simulink model "bh_solenoid_simscape_FINAL"  (R2018a)
settings: Solver=VariableStepAuto  StartTime=0.0  StopTime=3  MaxStep=0.01  RelTol=1e-3  AbsTol=1e-3  EnableMultiTasking=on
undefined symbols (not defined in the file): Coeffs, Elec, Mech, sigbuilder_block, solen
libraries: fl_lib x16, nesl_utility x7
CloseFcn:
  | try,close(h1_ssc_solenoid),end
  | clear h1_ssc_solenoid
  | 
  | clear simlog_ssc_solenoid
Description:
  | Solenoid
  | 
  | Copyright 2008-2017 The MathWorks, Inc.
settings Model: Creator=MathWorks  LastModifiedBy=bhorton
settings SolverCC: AutoScaleAbsTol=off
settings DataIOCC: LimitDataPoints=on  SaveFormat=Array
settings OptimizationCC: LifeSpan=inf
settings DebuggingCC: SolverPrmCheckMsg=warning  AllowSymbolicDim=off  SFUnexpectedBacktrackingDiag=warning  SFNoUnconditionalDefaultTransitionDiag=warning  SFExecutionAtInitializationDiag=none
settings HardwareCC: ProdBitPerPointer=32  ProdBitPerSizeT=32  ProdBitPerPtrDiffT=32  ProdLargestAtomicFloat=None  ProdIntDivRoundTo=Undefined  ProdEndianess=Unspecified  ProdWordSize=32  ProdHWDeviceType=32-bit Generic
settings ModelReferenceCC: PropagateSignalLabelsOutOfModel=off
settings CodeAppCC: StateflowObjectComments=on
settings GRTTargetCC: TargetLangStandard=C89/C90 (ANSI)  GeneratePreprocessorConditionals=Disable all
settings ConfigComp: CovMetricSettings=dw  CovHtmlReporting=on  CovSaveCumulativeToWorkspaceVar=on  CovSaveSingleToWorkspaceVar=on  CovExternalEMLEnable=off  CovSFcnEnable=off
settings SimscapeCC: SimscapeLogType=all  SimscapeLogSimulationStatistics=on  SimscapeLogName=simlog_ssc_solenoid  SimscapeLogDataHistory=10000

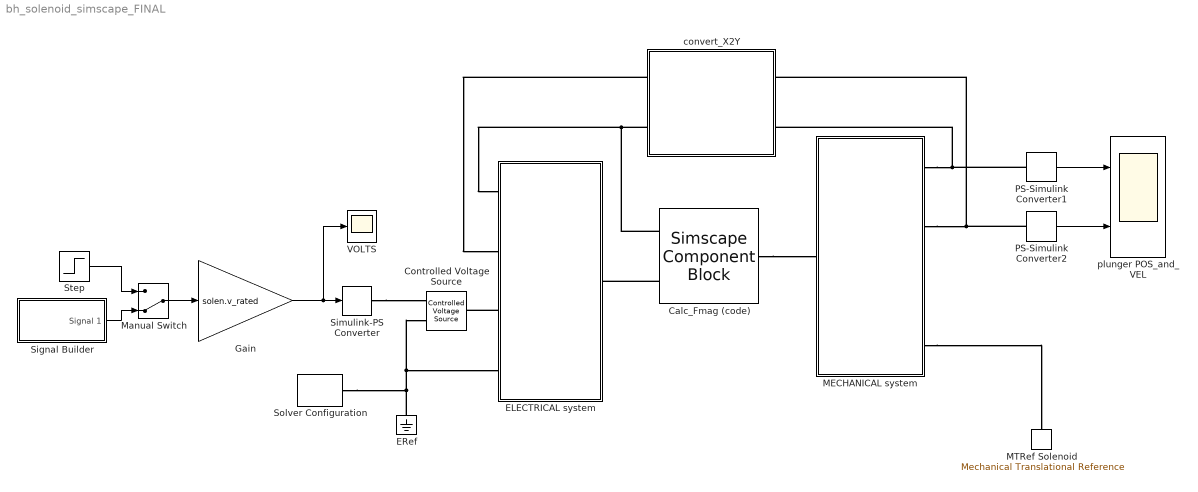
== system bh_solenoid_simscape_FINAL ==
  Calc_Fmag (code) : SimscapeComponentBlock  SourceFile=bh_Fmag  ComponentPath=bh_Fmag  ComponentVariants=bh_Fmag  ComponentVariantNames=bh_Fmag  ClassName=bh_Fmag  SchemaVersion=1  C1=Coeffs.C123(1) m^5*H  C2=Coeffs.C123(2) m^2  C3=Coeffs.C123(3) m^3
      settings: CopyFcn=simscape.engine.sli.internal.componentblockcallback(gcbh,'COPY')  PreCopyFcn=simscape.engine.sli.internal.componentblockcallback(gcbh,'PRECOPY')  PreDeleteFcn=simscape.engine.sli.internal.componentblockcallback(gcbh,'PREDELETE')
      mask Type: bh_Fmag
      mask Display:
      | disp('Simscape\n\n\n')
      | disp('\n\n\nbh_Fmag');
      | color('red');
      | port_label('RConn', 1,'Fmag');
      | port_label('LConn', 2,'i');
      | port_label('LConn', 1,'Y');
  Controlled Voltage Source : fl_lib/Electrical/Electrical Sources/Controlled Voltage Source
  ELECTRICAL system : Subsystem
  ERef : fl_lib/Electrical/Electrical Elements/Electrical Reference
  Gain : Gain  Gain=solen.v_rated
  MECHANICAL system : Subsystem
  MTRef Solenoid : fl_lib/Mechanical/Translational Elements/Mechanical Translational Reference
  Manual Switch : ManualSwitch  CurrentSetting=0
  PS-Simulink Converter1 : nesl_utility/PS-Simulink Converter  PhysicalDomain=network_engine_domain  SubClassName=ps_output  LeftPortType=input  RightPortType=output  PseudoPeriodic=off  Frequencies=[]  Unit=m  AffineConversion=off
      settings: AttributesFormatString=units=%<Unit>
  PS-Simulink Converter2 : nesl_utility/PS-Simulink Converter  PhysicalDomain=network_engine_domain  SubClassName=ps_output  LeftPortType=input  RightPortType=output  PseudoPeriodic=off  Frequencies=[]  Unit=m/s  AffineConversion=off
      settings: AttributesFormatString=units=%<Unit>
  Signal Builder : Subsystem  Tag=STV Subsys  LoadFcn=sigbuilder_block('load');  StartFcn=sigbuilder_block('start');  StopFcn=sigbuilder_block('stop');  ClipboardFcn=sigbuilder_block('clipboard');  mask(Sigbuilder block){tuvar=[0:10]}
      mask help: Simulink:masks:SigbuilderBlock_MD
      mask init:
      | if ~strcmp(get_param(bdroot(gcbh),'SimulationStatus'),'stopped') tuvar = sigbuilder_block('maskInit'); end
      settings: CopyFcn=sigbuilder_block('copy');  DeleteFcn=sigbuilder_block('delete');  ModelCloseFcn=sigbuilder_block('modelClose');  PreSaveFcn=sigbuilder_block('preSave');  PauseFcn=sigbuilder_block('pause');  ContinueFcn=sigbuilder_block('continue');  NameChangeFcn=sigbuilder_block('namechange');  OpenFcn=sigbuilder_block('open',[437.6 199.2 550.4 400 ]);  CloseFcn=sigbuilder_block('close');
      mask Display: plot(0, 0, 100, 100,[2, 2, 32, 32, 2], [68, 8, 8, 68, 68],[32, 2], [38, 38], [32, 19, 2],[53, 60, 44], [32, 17, 17, 2],[16, 16, 31, 31]);txt = getActiveGroup(gcbh);text(2, 100, txt,'verticalAlignment', 'top');
  Simulink-PS Converter : nesl_utility/Simulink-PS Converter  PhysicalDomain=network_engine_domain  SubClassName=ps_input  LeftPortType=input  RightPortType=output  PseudoPeriodic=off  Frequencies=[]  NoiseDistribution=none  NoiseParameters=[]  Unit=V  AffineConversion=off  FilteringAndDerivatives=provide  SimscapeFilterOrder=1  InputFilterTimeConstant=0.001  UdotUserProvided=0
  Solver Configuration : nesl_utility/Solver Configuration  PhysicalDomain=network_engine_domain  SubClassName=solver  LeftPortType=input  RightPortType=generic  Tones=[]  Harmonics=[]  SimulateNoise=off  Profile=off  UseLocalSampling=off  EnableSwitchedLinearOptims=on  FrequencyDomain=off  UseCCode=off  RelTol=0.001  AbsTol=1e-06  MinStep=1e-09  ToWorkspace=off  RevertToSquareIcSolve=off  NumHomotopyIterations=100  PhasorMode=off  PhasorModeNumHarmonics=1  DoDC=off  ResidualTolerance=1e-09  UseLocalSolver=off  LocalSolverChoice=NE_BACKWARD_EULER_ADVANCER  LocalSolverSampleTime=0.001  DoFixedCost=off  MaxNonlinIter=3  MaxModeIter=2  LinearAlgebra=Sparse  EquationFormulation=NE_TIME_EF  DelaysMemoryBudget=1024  AutomaticFiltering=on  FilteringTimeConstant=0.001
  Step : Step  Time=0.1  SampleTime=0
  VOLTS : Scope
  convert_X2Y : Subsystem
  plunger POS_and_VEL : Scope  NumInputPorts=2
  wires:
  Signal Builder/1(Signal 1) -> Manual Switch/2
  Manual Switch/1 -> Gain/1
  Step/1 -> Manual Switch/1
  Gain/1 -> VOLTS/1, Simulink-PS Converter/1
  PS-Simulink Converter1/1 -> plunger POS_and_VEL/1
  PS-Simulink Converter2/1 -> plunger POS_and_VEL/2
  connections:
  ELECTRICAL system/LConn3 -- Controlled Voltage Source/LConn1
  ERef/LConn1 -- Controlled Voltage Source/RConn2 -- ELECTRICAL system/LConn4 -- Solver Configuration/RConn1
  Simulink-PS Converter/RConn1 -- Controlled Voltage Source/RConn1
  MECHANICAL system/RConn1 -- PS-Simulink Converter1/LConn1 -- convert_X2Y/LConn2
  MECHANICAL system/RConn2 -- PS-Simulink Converter2/LConn1 -- convert_X2Y/LConn1
  convert_X2Y/RConn1 -- ELECTRICAL system/LConn2
  convert_X2Y/RConn2 -- Calc_Fmag (code)/LConn1 -- ELECTRICAL system/LConn1
  Calc_Fmag (code)/RConn1 -- MECHANICAL system/LConn1
  Calc_Fmag (code)/LConn2 -- ELECTRICAL system/RConn1
  MECHANICAL system/RConn4 -- MTRef Solenoid/LConn1

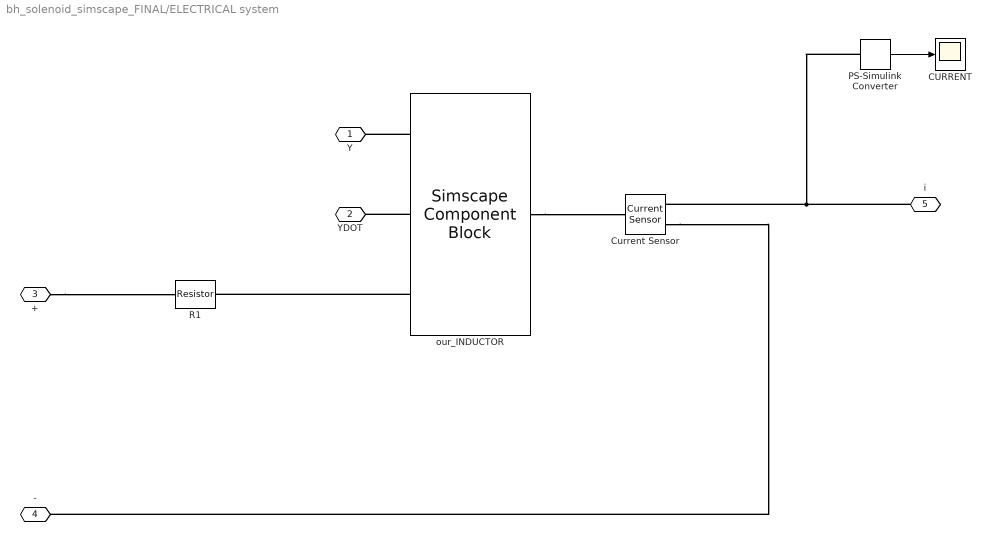
== system bh_solenoid_simscape_FINAL/ELECTRICAL system ==
  CURRENT : Scope
  Current Sensor : fl_lib/Electrical/Electrical Sensors/Current Sensor
  PS-Simulink Converter : nesl_utility/PS-Simulink Converter  PhysicalDomain=network_engine_domain  SubClassName=ps_output  LeftPortType=input  RightPortType=output  PseudoPeriodic=off  Frequencies=[]  Unit=A  AffineConversion=off
      settings: AttributesFormatString=unit=%<Unit>
  R1 : fl_lib/Electrical/Electrical Elements/Resistor  R=Elec.R Ohm  i_specify=off  i_priority=High  i=0 A  i_nominal_specify=off  i_nominal_unit=A  i_nominal_value=1  v_specify=off  v_priority=High  v=0 V  v_nominal_specify=off  v_nominal_unit=V  v_nominal_value=1
      settings: AttributesFormatString=R=%<R>
  our_INDUCTOR : SimscapeComponentBlock  SourceFile=bh_var_L  ComponentPath=bh_var_L  ComponentVariants=bh_var_L  ComponentVariantNames=bh_var_L  ClassName=bh_var_L  SchemaVersion=1  C1=Coeffs.C123(1) m^5*H  C2=Coeffs.C123(2) m^2  C3=Coeffs.C123(3) m^3  i_specify=off  i_priority=None  i=0 A  i_nominal_specify=off  i_nominal_unit=A  i_nominal_value=1  v_specify=off  v_priority=None  v=0 V  v_nominal_specify=off  v_nominal_unit=V  v_nominal_value=1
      settings: CopyFcn=simscape.engine.sli.internal.componentblockcallback(gcbh,'COPY')  PreCopyFcn=simscape.engine.sli.internal.componentblockcallback(gcbh,'PRECOPY')  PreDeleteFcn=simscape.engine.sli.internal.componentblockcallback(gcbh,'PREDELETE')
      mask Type: bh_var_L
      mask Display:
      | disp('Simscape\n\n\n')
      | disp('\n\n\nbh_var_L');
      | color('red');
      | port_label('RConn', 1,'-');
      | port_label('LConn', 3,'+');
      | port_label('LConn', 2,'Y_DOT');
      | port_label('LConn', 1,'Y');
  Y : PMIOPort  Side=Left
  YDOT : PMIOPort  Port=2  Side=Left
  + : PMIOPort  Port=3  Side=Left
  - : PMIOPort  Port=4  Side=Left
  i : PMIOPort  Port=5  Side=Right
  wires:
  PS-Simulink Converter/1 -> CURRENT/1
  connections:
  Current Sensor/RConn2 -- -/RConn1
  +/RConn1 -- R1/LConn1
  i/RConn1 -- PS-Simulink Converter/LConn1 -- Current Sensor/RConn1
  our_INDUCTOR/LConn1 -- Y/RConn1
  our_INDUCTOR/LConn2 -- YDOT/RConn1
  our_INDUCTOR/RConn1 -- Current Sensor/LConn1
  our_INDUCTOR/LConn3 -- R1/RConn1

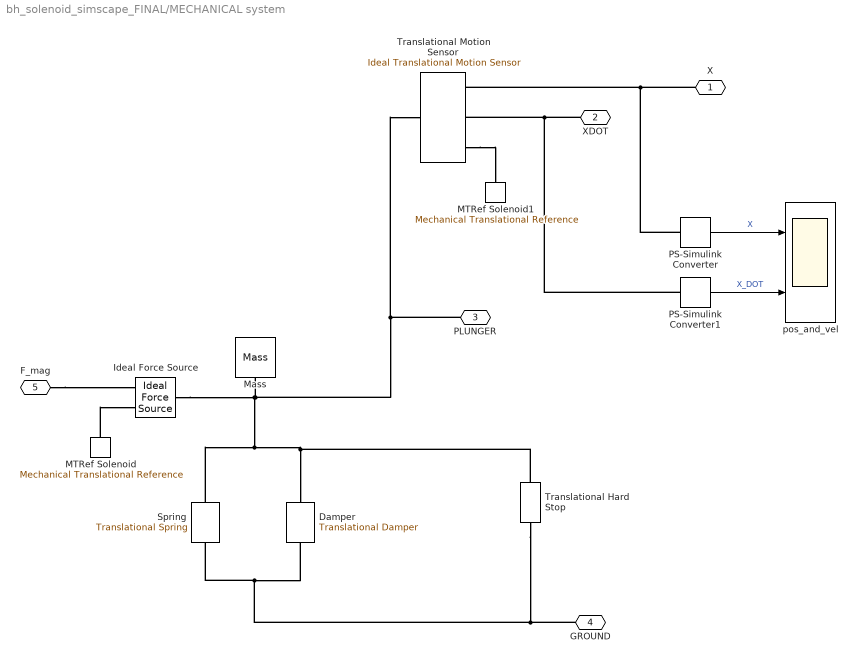
== system bh_solenoid_simscape_FINAL/MECHANICAL system ==
  Damper : fl_lib/Mechanical/Translational Elements/Translational Damper  D=Mech.C N/(m/s)  v_specify=off  v_priority=High  v=0 m/s  v_nominal_specify=off  v_nominal_unit=m/s  v_nominal_value=1  f_specify=off  f_priority=High  f=0 N  f_nominal_specify=off  f_nominal_unit=N  f_nominal_value=1
  Ideal Force Source : fl_lib/Mechanical/Mechanical Sources/Ideal Force Source
  MTRef Solenoid : fl_lib/Mechanical/Translational Elements/Mechanical Translational Reference
  MTRef Solenoid1 : fl_lib/Mechanical/Translational Elements/Mechanical Translational Reference
  Mass : fl_lib/Mechanical/Translational Elements/Mass  mass=Mech.M kg  v_specify=off  v_priority=High  v=0 m/s  v_nominal_specify=off  v_nominal_unit=m/s  v_nominal_value=1  f_specify=off  f_priority=High  f=0 N  f_nominal_specify=off  f_nominal_unit=N  f_nominal_value=1
  PS-Simulink Converter : nesl_utility/PS-Simulink Converter  PhysicalDomain=network_engine_domain  SubClassName=ps_output  LeftPortType=input  RightPortType=output  PseudoPeriodic=off  Frequencies=[]  Unit=m  AffineConversion=off
      settings: AttributesFormatString=unit=%<Unit>
  PS-Simulink Converter1 : nesl_utility/PS-Simulink Converter  PhysicalDomain=network_engine_domain  SubClassName=ps_output  LeftPortType=input  RightPortType=output  PseudoPeriodic=off  Frequencies=[]  Unit=m/s  AffineConversion=off
      settings: AttributesFormatString=unit=%<Unit>
  Spring : fl_lib/Mechanical/Translational Elements/Translational Spring  spr_rate=Mech.K N/m  v_specify=off  v_priority=High  v=0 m/s  v_nominal_specify=off  v_nominal_unit=m/s  v_nominal_value=1  f_specify=off  f_priority=High  f=0 N  f_nominal_specify=off  f_nominal_unit=N  f_nominal_value=1  x_specify=on  x_priority=High  x=Mech.x_0 m  x_nominal_specify=off  x_nominal_unit=m  x_nominal_value=1
      settings: AttributesFormatString=|
      | DEFLECTION=
      | %<x>
  Translational Motion Sensor : fl_lib/Mechanical/Mechanical Sensors/Ideal Translational Motion Sensor  offset=Mech.x_0 m
      settings: AttributesFormatString=|
      | init_VAL =
      | %<offset> %<offset_unit>
  Translational Hard Stop : fl_lib/Mechanical/Translational Elements/Translational Hard Stop  upper_bnd=Mech.x_max m  lower_bnd=Mech.x_min m  stiff_up=1e6 N/m  stiff_low=1e6 N/m  D_up=500 N/(m/s)  D_low=500 N/(m/s)  model=1  transition=0.1 mm  v_specify=off  v_priority=None  v=0 m/s  v_nominal_specify=off  v_nominal_unit=m/s  v_nominal_value=1  f_specify=off  f_priority=None  f=0 N  f_nominal_specify=off  f_nominal_unit=N  f_nominal_value=1  x_specify=off  x_priority=High  x=0 m  x_nominal_specify=off  x_nominal_unit=m  x_nominal_value=1
      settings: AttributesFormatString=|
      | LOWER_BND = %<lower_bnd>
      | UPPER_BND = %<upper_bnd>
  pos_and_vel : Scope  NumInputPorts=2
  X : PMIOPort  Side=Right
  XDOT : PMIOPort  Port=2  Side=Right
  PLUNGER : PMIOPort  Port=3  Side=Right
  GROUND : PMIOPort  Port=4  Side=Right
  F_mag : PMIOPort  Port=5  Side=Left
  wires:
  PS-Simulink Converter/1 -> pos_and_vel/1  "X"
  PS-Simulink Converter1/1 -> pos_and_vel/2  "X_DOT"
  connections:
  Damper/RConn1 -- Translational Hard Stop/RConn1 -- GROUND/RConn1 -- Spring/RConn1
  F_mag/RConn1 -- Ideal Force Source/RConn1
  MTRef Solenoid/LConn1 -- Ideal Force Source/RConn2
  Translational Motion Sensor/RConn1 -- MTRef Solenoid1/LConn1
  X/RConn1 -- PS-Simulink Converter/LConn1 -- Translational Motion Sensor/RConn3
  XDOT/RConn1 -- PS-Simulink Converter1/LConn1 -- Translational Motion Sensor/RConn2
  PLUNGER/RConn1 -- Translational Motion Sensor/LConn1 -- Translational Hard Stop/LConn1 -- Damper/LConn1 -- Spring/LConn1 -- Ideal Force Source/LConn1 -- Mass/LConn1

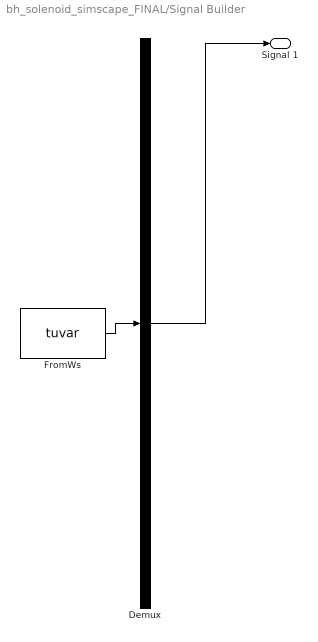
== system bh_solenoid_simscape_FINAL/Signal Builder ==
  Demux : Demux  Tag=STV Demux  Outputs=1
  FromWs : FromWorkspace  Tag=STV FromWs  VariableName=tuvar  SampleTime=0
      SigBuilderData=|
      | common.afterFinalStr = 'Extrapolate'
      | common.sampleTime = 0
      | dataSet.timeRange = [0 2]
      | dataSet.name = 'Group 1'
      | sbobj.Groups.Name = 'Group 1'
      | sbobj.Groups.Signals.Name = 'Signal 1'
      | sbobj.Groups.Signals.XData = [0 0.1 0.1 1.5 1.5 2]
      | sbobj.Groups.Signals.YData = [0 0 1 1 0 0]
      | sbobj.Groups.TimeRange = [0 2]
  Signal 1 : Outport  Tag=STV Outport
  wires:
  Demux/1 -> Signal 1/1
  FromWs/1 -> Demux/1

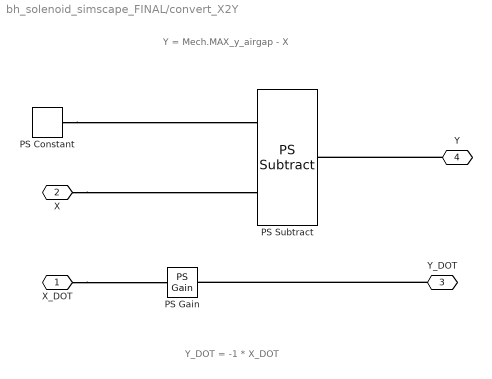
== system bh_solenoid_simscape_FINAL/convert_X2Y ==
  note: Y = Mech.MAX_y_airgap - X
  note: Y_DOT = -1 * X_DOT
  PS Constant : fl_lib/Physical Signals/Sources/PS Constant  constant=Mech.MAX_y_airgap
      settings: AttributesFormatString=%<constant>
  PS Gain : fl_lib/Physical Signals/Functions/PS Gain  gain=-1
      settings: AttributesFormatString=%<gain>
  PS Subtract : fl_lib/Physical Signals/Functions/PS Subtract
      settings: SourceProductName=Simscape
  X_DOT : PMIOPort  Side=Left
  X : PMIOPort  Port=2  Side=Left
  Y_DOT : PMIOPort  Port=3  Side=Right
  Y : PMIOPort  Port=4  Side=Right
  connections:
  PS Constant/RConn1 -- PS Subtract/LConn1
  X/RConn1 -- PS Subtract/LConn2
  Y/RConn1 -- PS Subtract/RConn1
  Y_DOT/RConn1 -- PS Gain/RConn1
  X_DOT/RConn1 -- PS Gain/LConn1
